simulink model "physicalModel"  (R2015b)
settings: Solver=VariableStepAuto  StartTime=0.0  StopTime=10.0  RelTol=1e-3
values from neighbouring files (symbols this model uses):
  c = 10    [main_physicalModel.m]    (also in main_plotsAndFigures.m = 2*sqrt(k*(1/m_m+1/m_l))*(m_m*m_l)/(m_m+m_l))
  D = 100    [main_physicalModel.m]
  k = 100    [main_physicalModel.m]    (also in main_plotsAndFigures.m = (1000:1:1000))
  m_l = 1    [main_physicalModel.m]    (also in main_plotsAndFigures.m)
  m_m = 1    [main_physicalModel.m]    (also in main_plotsAndFigures.m)
  P = 1000    [main_physicalModel.m]    (also in main_plotsAndFigures.m = -1000)
settings Model: Creator=atlas  LastModifiedBy=atlas

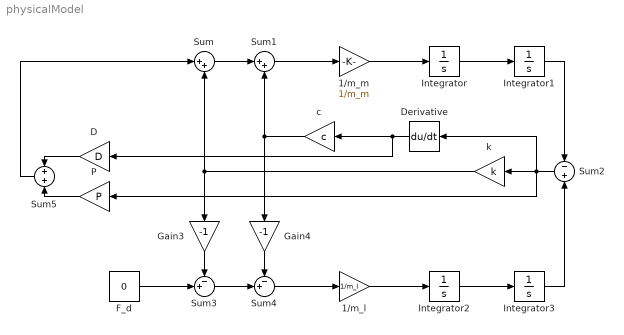
== system physicalModel ==
  1/m_l : Gain  Gain=1/m_l
  1/m_m : Gain  Gain=1/m_m
  D : Gain  Gain=D
  Derivative : Derivative
  F_d : Constant  Value=0
  Gain3 : Gain  Gain=-1
  Gain4 : Gain  Gain=-1
  Integrator{,1..3} (4 alike) : Integrator
  P : Gain  Gain=P
  Sum : Sum  Inputs=|++
  Sum1 : Sum  Inputs=|++
  Sum2 : Sum  Inputs=-+
  Sum3 : Sum  Inputs=-+|
  Sum4 : Sum  Inputs=-+|
  Sum5 : Sum
  c : Gain  Gain=c
  k : Gain  Gain=k
  wires:
  Sum5/1 -> Sum/1
  Sum/1 -> Sum1/1
  Sum1/1 -> 1/m_m/1
  1/m_m/1 -> Integrator/1
  Integrator/1 -> Integrator1/1
  Integrator1/1 -> Sum2/1
  Sum4/1 -> 1/m_l/1
  1/m_l/1 -> Integrator2/1
  Integrator2/1 -> Integrator3/1
  Integrator3/1 -> Sum2/2
  Sum2/1 -> P/1, Derivative/1, k/1
  k/1 -> Sum/2, Gain3/1
  F_d/1 -> Sum3/2
  Gain3/1 -> Sum3/1
  Sum3/1 -> Sum4/2
  Derivative/1 -> D/1, c/1
  Gain4/1 -> Sum4/1
  c/1 -> Sum1/2, Gain4/1
  P/1 -> Sum5/2
  D/1 -> Sum5/1
